simulink model "PS_HVAC19_prev"  (R2023b)
settings: Solver=FixedStepAuto  StartTime=0.0  StopTime=inf  RelTol=1e-3  AbsTol=1e-6
model workspace (MATLAB code in the model file + MAT data in the model file):
  LWall = 0.2
  LWindow = 0.01
  M = 1778.36911446
  Mdot = 3600
  PLC_IP_Address = 'localhost'
  RWall = 1.52148180317e-06
  RWindow = 5.93542260209e-07
  Req = 4.26975637751e-07
  THeater = 50
  TinIC = 20
  c = 1005.4
  cost = 2.5e-08
  densAir = 1.225
  htHouse = 4
  htWindows = 1
  kWall = 136.8
  kWindow = 2808
  lenHouse = 30
  numWindows = 6
  pitRoof = 0.698131700798
  r2d = 57.2957795131
  wallArea = 960.897659797
  widHouse = 10
  widWindows = 1
  windowArea = 6
  other statements: sldemo_househeat_data
libraries: dspnetwork x20, simulink_extras x2
Description:
  | Thermal Model of a House
  | 
  | This demo illustrates how you can use Simulink(R) to create the thermal model of
  | a house. This system models the outdoor environment, the thermal
  | characteristics of the house, and the house heating system.
  | 
  | The sldemo_househeat_data.m file initializes data in the model workspace.
  | To make changes, you can edit the model workspace directly or edit the MATLAB(R) file
  | and re-load the model workspace.
  | 
  | To view the model workspace, select View > Model Explorer
  | from the Simulink editor.
  | 
  | Note: Time is given in units of hours
settings Model: Creator=The MathWorks, Inc.  LastModifiedBy=chase
settings SolverCC: AutoScaleAbsTol=off  AlgebraicLoopSolver=TrustRegion
settings DataIOCC: ExternalInput=[]  InitialState=[]  SaveFormat=Array  SaveOutput=off  SaveTime=off  ReturnWorkspaceOutputs=off  SignalLoggingName=sldemo_househeat_output
settings OptimizationCC: BlockReduction=off  BooleanDataType=off  ExpressionDepthLimit=2147483647  InitFltsAndDblsToZero=on  LifeSpan=inf  BufferReusableBoundary=off
settings DebuggingCC: SaveWithParameterizedLinksMsg=none  UnderspecifiedInitializationDetection=Classic  MergeDetectMultiDrivingBlocksExec=none  SignalResolutionControl=TryResolveAllWithWarning  MultiTaskDSMMsg=warning  MultiTaskCondExecSysMsg=none  IntegerOverflowMsg=none  FcnCallInpInsideContextMsg=warning  UnconnectedInputMsg=warning  UnconnectedOutputMsg=warning  UnconnectedLineMsg=warning  BusObjectLabelMismatch=none  StateNameClashWarn=warning  SFUnexpectedBacktrackingDiag=warning  SFNoUnconditionalDefaultTransitionDiag=warning  SFExecutionAtInitializationDiag=none  IntegerSaturationMsg=none  ArithmeticOperatorsInVariantConditions=warning
settings HardwareCC: ProdBitPerPointer=32  ProdBitPerSizeT=32  ProdBitPerPtrDiffT=32  ProdLargestAtomicFloat=None  ProdIntDivRoundTo=Undefined  ProdEndianess=Unspecified  ProdWordSize=32  ProdHWDeviceType=32-bit Generic  TargetBitPerPointer=64  TargetBitPerSizeT=64  TargetBitPerPtrDiffT=64  TargetLongLongMode=on  TargetIntDivRoundTo=Zero  TargetEndianess=LittleEndian  TargetWordSize=64  TargetHWDeviceType=MATLAB Host  ProdEqTarget=off
settings ModelReferenceCC: EnableRefExpFcnMdlSchedulingChecks=on  PropagateSignalLabelsOutOfModel=off
settings SFSimCC: SimUseLocalCustomCode=off  CustomCodeUndefinedFunction=UseInterfaceOnly
settings RTWCC: PackageGeneratedCodeAndArtifacts=on  PackageName=HVAC  RTWUseLocalCustomCode=off
settings CodeAppCC: StateflowObjectComments=on
settings GRTTargetCC: TargetFcnLib=ansi_tfl_tmw.mat  TargetLangStandard=C89/C90 (ANSI)  CombineOutputUpdateFcns=off  GRTInterface=on
settings ConfigComp: CovMetricSettings=dw  CovSaveCumulativeToWorkspaceVar=on  CovSaveSingleToWorkspaceVar=on  CovExternalEMLEnable=off

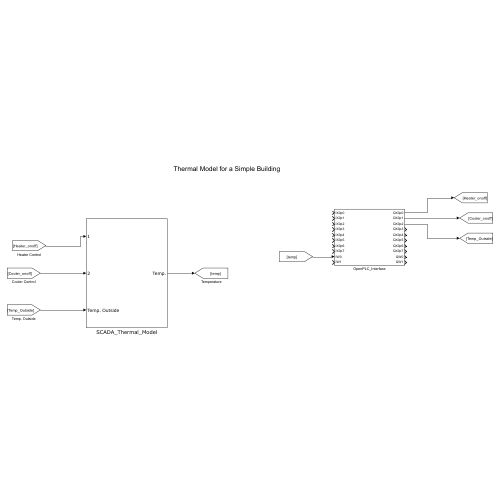
[thumbnail: Simulink's stored preview of the top-level diagram]
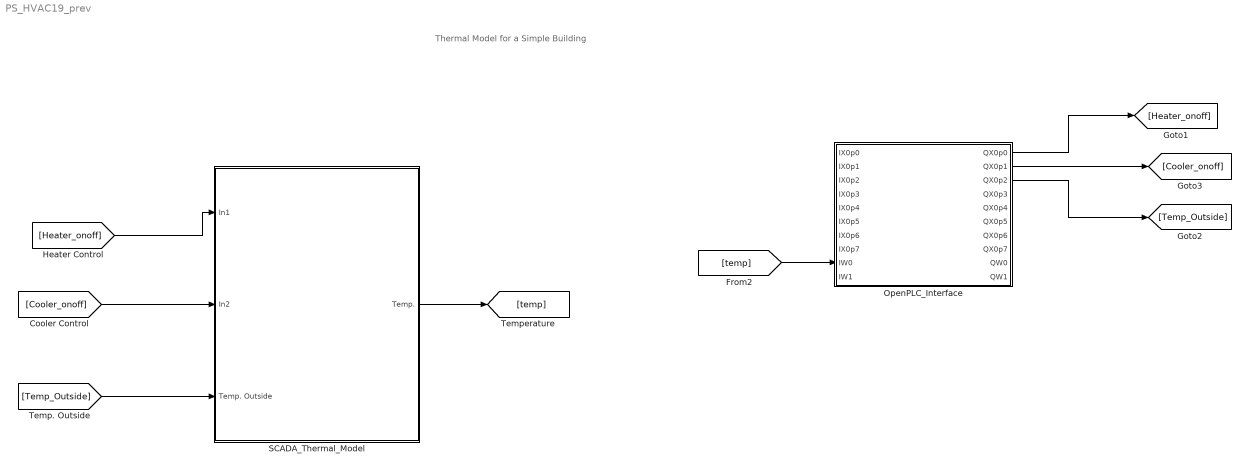
== system PS_HVAC19_prev ==
  note: Thermal Model for a Simple Building
  OpenPLC_Interface : Subsystem
  SCADA_Thermal_Model : Subsystem
  wires:
  SCADA_Thermal_Model/1(Temp.) -> [temp]
  [temp] -> OpenPLC_Interface/9(IW0)
  [Heater_onoff] -> SCADA_Thermal_Model/1(In1)
  [Cooler_onoff] -> SCADA_Thermal_Model/2(In2)
  OpenPLC_Interface/1(QX0p0) -> [Heater_onoff]
  OpenPLC_Interface/2(QX0p1) -> [Cooler_onoff]
  [Temp_Outside] -> SCADA_Thermal_Model/3(Temp. Outside)
  OpenPLC_Interface/3(QX0p2) -> [Temp_Outside]

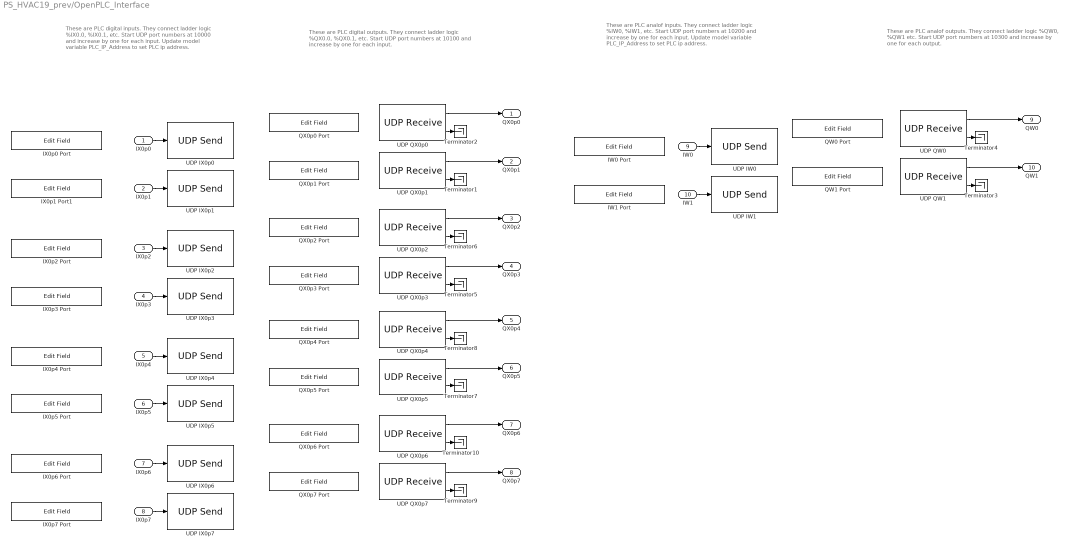
== system PS_HVAC19_prev/OpenPLC_Interface ==
  note: These are PLC digital inputs. They connect
      | ladder logic %IX0.0, %IX0.1, etc.
      |
      | Start UDP port numbers at 10000 and
      | increase by one for each input.
      |
      | Update model variable PLC_IP_Address
      | to set PLC ip address.
  note: These are PLC digital outputs. They connect
      | ladder logic %QX0.0, %QX0.1, etc.
      |
      | Start UDP port numbers at 10100 and increase
      | by one for each input.
  note: These are PLC analof inputs. They connect
      | ladder logic %IW0, %IW1, etc.
      |
      | Start UDP port numbers  at 10200 and
      | increase by one for each input.
      |
      | Update model variable PLC_IP_Address
      | to set PLC ip address.
  note: These are PLC analof outputs. They connect
      | ladder logic %QW0, %QW1 etc.
      |
      | Start UDP port numbers at 10300 and increase
      | by one for each output.
  "IX0p0 " : Inport
  IX0p1 : Inport  Port=2
  IX0p2 : Inport  Port=3
  IX0p3 : Inport  Port=4
  IX0p4 : Inport  Port=5
  IX0p5 : Inport  Port=6
  IX0p6 : Inport  Port=7
  IX0p7 : Inport  Port=8
  IW0 : Inport  Port=9
  IW1 : Inport  Port=10
  IW0 Port : EditField  LabelPosition=Hide  ShowInitialText=on  Alignment=Center
  IW1 Port : EditField  LabelPosition=Hide  ShowInitialText=on  Alignment=Center
  IX0p0 Port : EditField  LabelPosition=Hide  ShowInitialText=on  Alignment=Center
  IX0p1 Port1 : EditField  LabelPosition=Hide  ShowInitialText=on  Alignment=Center
  IX0p2 Port : EditField  LabelPosition=Hide  ShowInitialText=on  Alignment=Center
  IX0p3 Port : EditField  LabelPosition=Hide  ShowInitialText=on  Alignment=Center
  IX0p4 Port : EditField  LabelPosition=Hide  ShowInitialText=on  Alignment=Center
  IX0p5 Port : EditField  LabelPosition=Hide  ShowInitialText=on  Alignment=Center
  IX0p6 Port : EditField  LabelPosition=Hide  ShowInitialText=on  Alignment=Center
  IX0p7 Port : EditField  LabelPosition=Hide  ShowInitialText=on  Alignment=Center
  QW0 Port : EditField  LabelPosition=Hide  ShowInitialText=on  Alignment=Center
  QW1 Port : EditField  LabelPosition=Hide  ShowInitialText=on  Alignment=Center
  QX0p0 Port : EditField  LabelPosition=Hide  ShowInitialText=on  Alignment=Center
  QX0p1 Port : EditField  LabelPosition=Hide  ShowInitialText=on  Alignment=Center
  QX0p2 Port : EditField  LabelPosition=Hide  ShowInitialText=on  Alignment=Center
  QX0p3 Port : EditField  LabelPosition=Hide  ShowInitialText=on  Alignment=Center
  QX0p4 Port : EditField  LabelPosition=Hide  ShowInitialText=on  Alignment=Center
  QX0p5 Port : EditField  LabelPosition=Hide  ShowInitialText=on  Alignment=Center
  QX0p6 Port : EditField  LabelPosition=Hide  ShowInitialText=on  Alignment=Center
  QX0p7 Port : EditField  LabelPosition=Hide  ShowInitialText=on  Alignment=Center
  Terminator{1..10} (10 alike) : Terminator
  UDP IW0 : dspnetwork/UDP Send  remoteURL='localhost'  remotePort=10200  localURL='255.255.255.255'  localPortSource=Automatically determine  localPort=-1  sendBufferSize=8192  sampletime=-1  blockPlatform=LINUX  separateLengthPort=0
  UDP IW1 : dspnetwork/UDP Send  remoteURL='localhost'  remotePort=10201  localURL='255.255.255.255'  localPortSource=Automatically determine  localPort=-1  sendBufferSize=8192  sampletime=-1  blockPlatform=LINUX  separateLengthPort=0
  UDP IX0p0 : dspnetwork/UDP Send  remoteURL='localhost'  remotePort=10000  localURL='255.255.255.255'  localPortSource=Automatically determine  localPort=-1  sendBufferSize=8192  sampletime=-1  blockPlatform=LINUX  separateLengthPort=0
  UDP IX0p1 : dspnetwork/UDP Send  remoteURL='localhost'  remotePort=10001  localURL='255.255.255.255'  localPortSource=Automatically determine  localPort=-1  sendBufferSize=8192  sampletime=-1  blockPlatform=LINUX  separateLengthPort=0
  UDP IX0p2 : dspnetwork/UDP Send  remoteURL='localhost'  remotePort=10002  localURL='255.255.255.255'  localPortSource=Automatically determine  localPort=-1  sendBufferSize=8192  sampletime=-1  blockPlatform=LINUX  separateLengthPort=0
  UDP IX0p3 : dspnetwork/UDP Send  remoteURL='localhost'  remotePort=10003  localURL='255.255.255.255'  localPortSource=Automatically determine  localPort=-1  sendBufferSize=8192  sampletime=-1  blockPlatform=LINUX  separateLengthPort=0
  UDP IX0p4 : dspnetwork/UDP Send  remoteURL='localhost'  remotePort=10004  localURL='255.255.255.255'  localPortSource=Automatically determine  localPort=-1  sendBufferSize=8192  sampletime=-1  blockPlatform=LINUX  separateLengthPort=0
  UDP IX0p5 : dspnetwork/UDP Send  remoteURL='localhost'  remotePort=10005  localURL='255.255.255.255'  localPortSource=Automatically determine  localPort=-1  sendBufferSize=8192  sampletime=-1  blockPlatform=LINUX  separateLengthPort=0
  UDP IX0p6 : dspnetwork/UDP Send  remoteURL='localhost'  remotePort=10006  localURL='255.255.255.255'  localPortSource=Automatically determine  localPort=-1  sendBufferSize=8192  sampletime=-1  blockPlatform=LINUX  separateLengthPort=0
  UDP IX0p7 : dspnetwork/UDP Send  remoteURL='localhost'  remotePort=10007  localURL='255.255.255.255'  localPortSource=Automatically determine  localPort=-1  sendBufferSize=8192  sampletime=-1  blockPlatform=LINUX  separateLengthPort=0
  UDP QW0 : dspnetwork/UDP Receive  localURL='0.0.0.0'  localPort=10300  remoteURL='0.0.0.0'  remotePort=-1  recvBufferSize=2  dims=1  signalDatatype=uint16  isComplex=off  isVarSize=off  showBlockingTime=on  blockingTime=0  sampletime=0.01  blockPlatform=LINUX
  UDP QW1 : dspnetwork/UDP Receive  localURL='0.0.0.0'  localPort=10301  remoteURL='0.0.0.0'  remotePort=-1  recvBufferSize=2  dims=1  signalDatatype=uint16  isComplex=off  isVarSize=off  showBlockingTime=on  blockingTime=0  sampletime=0.01  blockPlatform=LINUX
  UDP QX0p0 : dspnetwork/UDP Receive  localURL='0.0.0.0'  localPort=10100  remoteURL='0.0.0.0'  remotePort=-1  recvBufferSize=2  dims=1  signalDatatype=uint16  isComplex=off  isVarSize=off  showBlockingTime=on  blockingTime=0  sampletime=0.01  blockPlatform=LINUX
  UDP QX0p1 : dspnetwork/UDP Receive  localURL='0.0.0.0'  localPort=10101  remoteURL='0.0.0.0'  remotePort=-1  recvBufferSize=2  dims=1  signalDatatype=uint16  isComplex=off  isVarSize=off  showBlockingTime=on  blockingTime=0  sampletime=0.01  blockPlatform=LINUX
  UDP QX0p2 : dspnetwork/UDP Receive  localURL='0.0.0.0'  localPort=10102  remoteURL='0.0.0.0'  remotePort=-1  recvBufferSize=2  dims=1  signalDatatype=uint16  isComplex=off  isVarSize=off  showBlockingTime=on  blockingTime=0  sampletime=0.01  blockPlatform=LINUX
  UDP QX0p3 : dspnetwork/UDP Receive  localURL='0.0.0.0'  localPort=10103  remoteURL='0.0.0.0'  remotePort=-1  recvBufferSize=2  dims=1  signalDatatype=uint16  isComplex=off  isVarSize=off  showBlockingTime=on  blockingTime=0  sampletime=0.01  blockPlatform=LINUX
  UDP QX0p4 : dspnetwork/UDP Receive  localURL='0.0.0.0'  localPort=10104  remoteURL='0.0.0.0'  remotePort=-1  recvBufferSize=2  dims=1  signalDatatype=uint16  isComplex=off  isVarSize=off  showBlockingTime=on  blockingTime=0  sampletime=0.01  blockPlatform=LINUX
  UDP QX0p5 : dspnetwork/UDP Receive  localURL='0.0.0.0'  localPort=10105  remoteURL='0.0.0.0'  remotePort=-1  recvBufferSize=2  dims=1  signalDatatype=uint16  isComplex=off  isVarSize=off  showBlockingTime=on  blockingTime=0  sampletime=0.01  blockPlatform=LINUX
  UDP QX0p6 : dspnetwork/UDP Receive  localURL='0.0.0.0'  localPort=10106  remoteURL='0.0.0.0'  remotePort=-1  recvBufferSize=2  dims=1  signalDatatype=uint16  isComplex=off  isVarSize=off  showBlockingTime=on  blockingTime=0  sampletime=0.01  blockPlatform=LINUX
  UDP QX0p7 : dspnetwork/UDP Receive  localURL='0.0.0.0'  localPort=10107  remoteURL='0.0.0.0'  remotePort=-1  recvBufferSize=2  dims=1  signalDatatype=uint16  isComplex=off  isVarSize=off  showBlockingTime=on  blockingTime=0  sampletime=0.01  blockPlatform=LINUX
  QX0p0 : Outport
  QX0p1 : Outport  Port=2
  QX0p2 : Outport  Port=3
  QX0p3 : Outport  Port=4
  QX0p4 : Outport  Port=5
  QX0p5 : Outport  Port=6
  QX0p6 : Outport  Port=7
  QX0p7 : Outport  Port=8
  QW0 : Outport  Port=9
  QW1 : Outport  Port=10
  wires:
  IX0p1/1 -> UDP IX0p1/1
  "IX0p0 "/1 -> UDP IX0p0/1
  UDP QX0p0/1 -> QX0p0/1
  UDP QX0p0/2 -> Terminator2/1
  UDP QX0p1/2 -> Terminator1/1
  UDP QX0p1/1 -> QX0p1/1
  IW1/1 -> UDP IW1/1
  IW0/1 -> UDP IW0/1
  UDP QW1/1 -> QW1/1
  UDP QW1/2 -> Terminator3/1
  UDP QW0/2 -> Terminator4/1
  UDP QW0/1 -> QW0/1
  IX0p2/1 -> UDP IX0p2/1
  IX0p3/1 -> UDP IX0p3/1
  IX0p7/1 -> UDP IX0p7/1
  IX0p6/1 -> UDP IX0p6/1
  IX0p4/1 -> UDP IX0p4/1
  IX0p5/1 -> UDP IX0p5/1
  UDP QX0p2/1 -> QX0p2/1
  UDP QX0p2/2 -> Terminator6/1
  UDP QX0p3/1 -> QX0p3/1
  UDP QX0p3/2 -> Terminator5/1
  UDP QX0p7/2 -> Terminator9/1
  UDP QX0p7/1 -> QX0p7/1
  UDP QX0p6/1 -> QX0p6/1
  UDP QX0p6/2 -> Terminator10/1
  UDP QX0p4/1 -> QX0p4/1
  UDP QX0p4/2 -> Terminator8/1
  UDP QX0p5/1 -> QX0p5/1
  UDP QX0p5/2 -> Terminator7/1

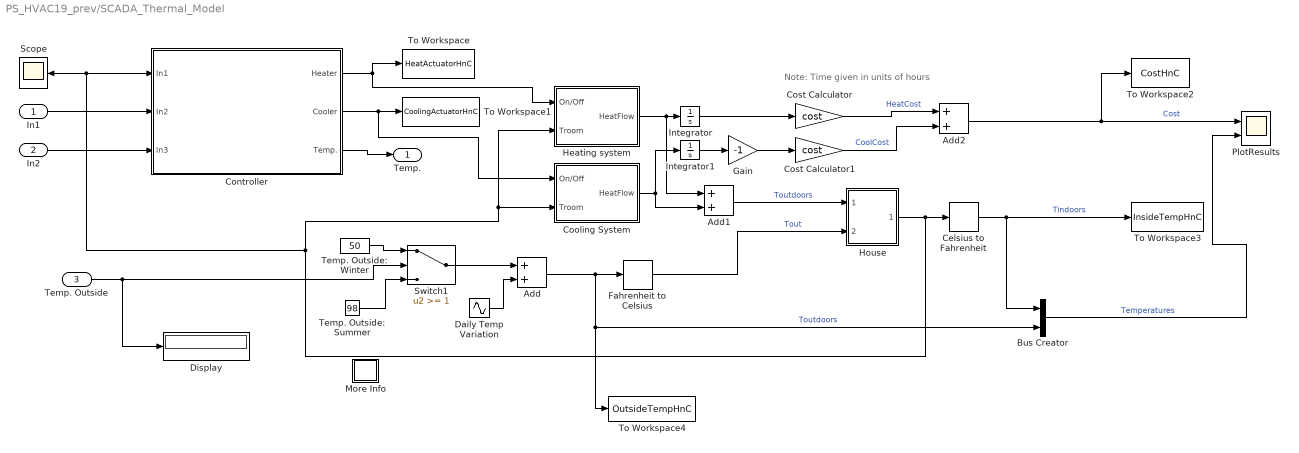
== system PS_HVAC19_prev/SCADA_Thermal_Model ==
  note: Note: Time given in units of hours
  In1 : Inport
  In2 : Inport  Port=2
  Temp. Outside : Inport  Port=3
  Add : Sum
  Add1 : Sum
  Add2 : Sum
  Bus Creator : BusCreator  Inputs=2
  Celsius to Fahrenheit : simulink_extras/Transformations/Celsius to Fahrenheit
  Controller : Subsystem
  Cooling System : Subsystem
  Cost Calculator : Gain  Gain=cost  SaturateOnIntegerOverflow=on  OutDataTypeStr=Inherit: Same as input  ParamDataTypeStr=Inherit: Same as input
  Cost Calculator1 : Gain  Gain=cost  SaturateOnIntegerOverflow=on  OutDataTypeStr=Inherit: Same as input  ParamDataTypeStr=Inherit: Same as input
  Daily Temp Variation : Sin  Frequency=2*pi/24  SampleTime=0
  Display : Display
  Fahrenheit to Celsius : simulink_extras/Transformations/Fahrenheit to Celsius
  Gain : Gain  Gain=-1
  Heating system : Subsystem
  House : Subsystem
      mask Display: image(fullfile(matlabroot,'toolbox','simulink','simdemos','simgeneral','images','HouseHeatHousePix.svg'))
  Integrator : Integrator
  Integrator1 : Integrator
  More Info : Subsystem
      settings: OpenFcn=showExample('simulink_general/sldemo_househeatExample')
      mask Display: disp('?')
  PlotResults : Scope  NumInputPorts=2
  Scope : Scope
  Switch1 : Switch  Threshold=1  SaturateOnIntegerOverflow=off  InputSameDT=off
  Temp. Outside: Summer : Constant  Value=98
  Temp. Outside: Winter : Constant  Value=50
  To Workspace : ToWorkspace  VariableName=HeatActuatorHnC  SaveFormat=Timeseries  SampleTime=.005
  To Workspace1 : ToWorkspace  VariableName=CoolingActuatorHnC  SaveFormat=Timeseries  SampleTime=.005
  To Workspace2 : ToWorkspace  VariableName=CostHnC  SaveFormat=Timeseries  SampleTime=.005
  To Workspace3 : ToWorkspace  VariableName=InsideTempHnC  SaveFormat=Timeseries  SampleTime=.005
  To Workspace4 : ToWorkspace  VariableName=OutsideTempHnC  SaveFormat=Timeseries  SampleTime=.005
  Temp. : Outport  VectorParamsAs1DForOutWhenUnconnected=off
  wires:
  Celsius to Fahrenheit/1 -> To Workspace3/1, Bus Creator/1  "Tindoors"
  Add/1 -> To Workspace4/1, Bus Creator/2, Fahrenheit to Celsius/1  "Toutdoors"
  Controller/1(Heater) -> Heating system/1(On/Off), To Workspace/1
  Cost Calculator/1 -> Add2/1  "HeatCost"
  Integrator1/1 -> Gain/1
  Heating system/1(HeatFlow) -> Add1/1, Integrator/1
  Cooling System/1(HeatFlow) -> Add1/2, Integrator1/1
  Add2/1 -> To Workspace2/1, PlotResults/1  "Cost"
  Daily Temp Variation/1 -> Add/2
  Add1/1 -> House/1(Heater QDot In)  "Toutdoors"
  Bus Creator/1 -> PlotResults/2  "Temperatures"
  Integrator/1 -> Cost Calculator/1
  Cost Calculator1/1 -> Add2/2  "CoolCost"
  Controller/2(Cooler) -> Cooling System/1(On/Off), To Workspace1/1
  Gain/1 -> Cost Calculator1/1
  Fahrenheit to Celsius/1 -> House/2(Outdoor Temp Tout)  "Tout"
  Controller/3(Temp.) -> Temp./1
  House/1(Room Temp Troom) -> Heating system/2(Troom), Cooling System/2(Troom), Scope/1, Controller/1(In1), Celsius to Fahrenheit/1
  In1/1 -> Controller/2(In2)
  In2/1 -> Controller/3(In3)
  Temp. Outside/1 -> Display/1, Switch1/2
  Temp. Outside: Winter/1 -> Switch1/1
  Temp. Outside: Summer/1 -> Switch1/3
  Switch1/1 -> Add/1

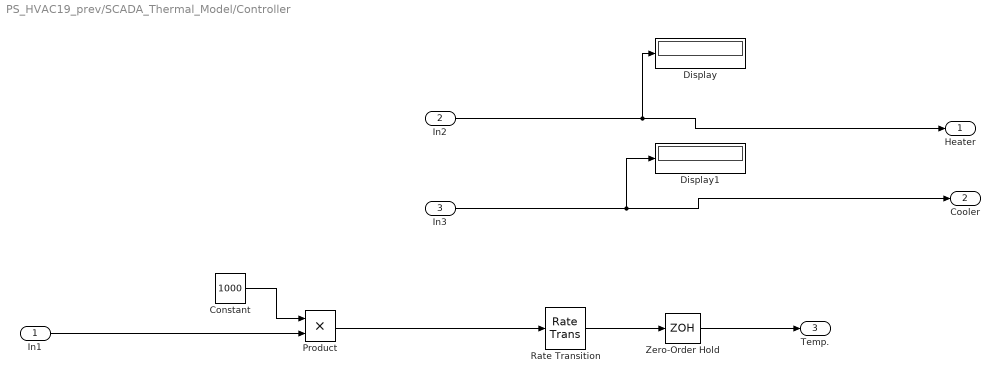
== system PS_HVAC19_prev/SCADA_Thermal_Model/Controller ==
  In1 : Inport
  In2 : Inport  Port=2
  In3 : Inport  Port=3
  Constant : Constant  Value=1000
  Display : Display
  Display1 : Display
  Product : Product
  Rate Transition : RateTransition
  Zero-Order Hold : ZeroOrderHold  SampleTime=0.005
  Heater : Outport  VectorParamsAs1DForOutWhenUnconnected=off
  Cooler : Outport  Port=2  VectorParamsAs1DForOutWhenUnconnected=off
  Temp. : Outport  Port=3  VectorParamsAs1DForOutWhenUnconnected=off
  wires:
  Constant/1 -> Product/1
  In1/1 -> Product/2
  Rate Transition/1 -> Zero-Order Hold/1
  Product/1 -> Rate Transition/1
  Zero-Order Hold/1 -> Temp./1
  In2/1 -> Display/1, Heater/1
  In3/1 -> Display1/1, Cooler/1

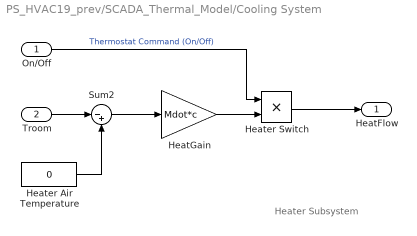
== system PS_HVAC19_prev/SCADA_Thermal_Model/Cooling System ==
  note: Heater Subsystem
  On/Off : Inport
  Troom : Inport  Port=2
  HeatGain : Gain  Gain=Mdot*c
  Heater Air Temperature : Constant  Value=0
  Heater Switch : Product  RndMeth=Zero
  Sum2 : Sum  Inputs=|-+
  HeatFlow : Outport  VectorParamsAs1DForOutWhenUnconnected=off
  wires:
  Heater Air Temperature/1 -> Sum2/2
  Troom/1 -> Sum2/1
  Sum2/1 -> HeatGain/1
  On/Off/1 -> Heater Switch/1  "Thermostat Command (On/Off)"
  HeatGain/1 -> Heater Switch/2
  Heater Switch/1 -> HeatFlow/1

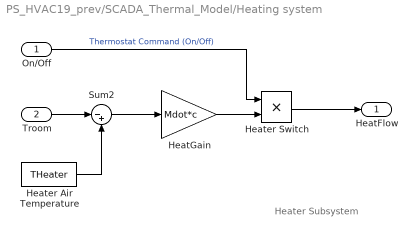
== system PS_HVAC19_prev/SCADA_Thermal_Model/Heating system ==
  note: Heater Subsystem
  On/Off : Inport
  Troom : Inport  Port=2
  HeatGain : Gain  Gain=Mdot*c
  Heater Air Temperature : Constant  Value=THeater
  Heater Switch : Product  RndMeth=Zero
  Sum2 : Sum  Inputs=|-+
  HeatFlow : Outport  VectorParamsAs1DForOutWhenUnconnected=off
  wires:
  Heater Air Temperature/1 -> Sum2/2
  Troom/1 -> Sum2/1
  Sum2/1 -> HeatGain/1
  On/Off/1 -> Heater Switch/1  "Thermostat Command (On/Off)"
  HeatGain/1 -> Heater Switch/2
  Heater Switch/1 -> HeatFlow/1

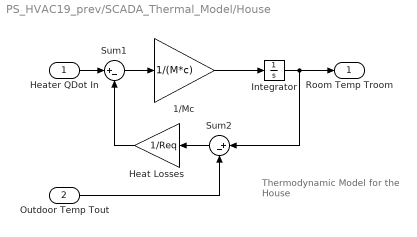
== system PS_HVAC19_prev/SCADA_Thermal_Model/House ==
  note: Thermodynamic Model
      | for the House
  Heater QDot In : Inport
  Outdoor Temp Tout : Inport  Port=2
  1/Mc : Gain  Gain=1/(M*c)  SaturateOnIntegerOverflow=on  OutDataTypeStr=Inherit: Same as input  ParamDataTypeStr=Inherit: Same as input
  Heat Losses : Gain  Gain=1/Req  SaturateOnIntegerOverflow=on  OutDataTypeStr=Inherit: Same as input  ParamDataTypeStr=Inherit: Same as input
  Integrator : Integrator  InitialCondition=TinIC
  Sum1 : Sum  Inputs=|+-  InputSameDT=on  SaturateOnIntegerOverflow=on  OutDataTypeStr=Inherit: Same as first input
  Sum2 : Sum  Inputs=|+-  InputSameDT=on  SaturateOnIntegerOverflow=on  OutDataTypeStr=Inherit: Same as first input
  Room Temp Troom : Outport  InitialOutput=0  VectorParamsAs1DForOutWhenUnconnected=off
  wires:
  Outdoor Temp Tout/1 -> Sum2/2
  Heater QDot In/1 -> Sum1/1
  Sum1/1 -> 1/Mc/1
  Sum2/1 -> Heat Losses/1
  Heat Losses/1 -> Sum1/2
  1/Mc/1 -> Integrator/1
  Integrator/1 -> Sum2/1, Room Temp Troom/1

== system PS_HVAC19_prev/SCADA_Thermal_Model/More Info ==
